simulink model "temperature"  (R2022a)
settings: Solver=VariableStepAuto  StartTime=0.0  StopTime=10.0  RelTol=1e-3
libraries: simulink x2, simulink_extras x1
settings Model: Creator=CTEA  LastModifiedBy=CTEA

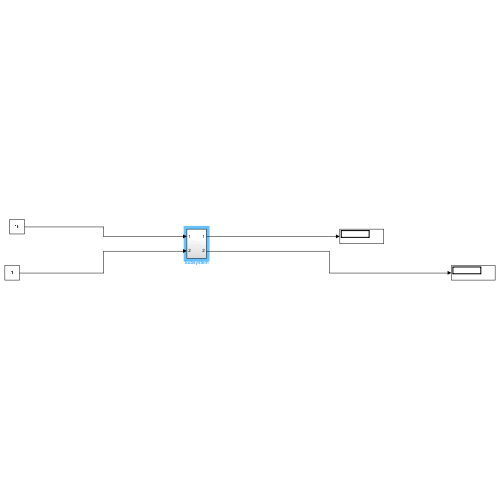
[thumbnail: Simulink's stored preview of the top-level diagram]
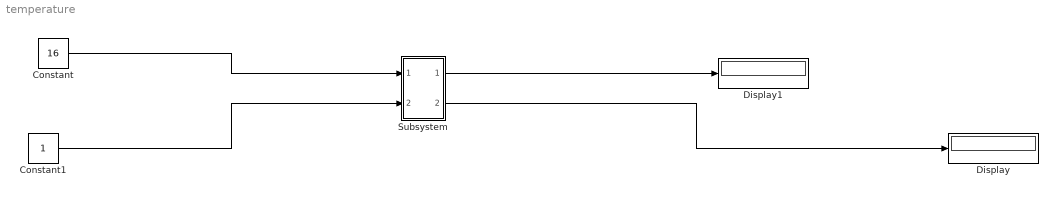
== system temperature ==
  Constant : Constant  Value=16  VectorParams1D=off
  Constant1 : Constant
  Display : Display
  Display1 : Display
  Subsystem : Subsystem
  wires:
  Constant/1 -> Subsystem/1(In1)
  Constant1/1 -> Subsystem/2(In2)
  Subsystem/2(Out1) -> Display/1
  Subsystem/1(Out2) -> Display1/1

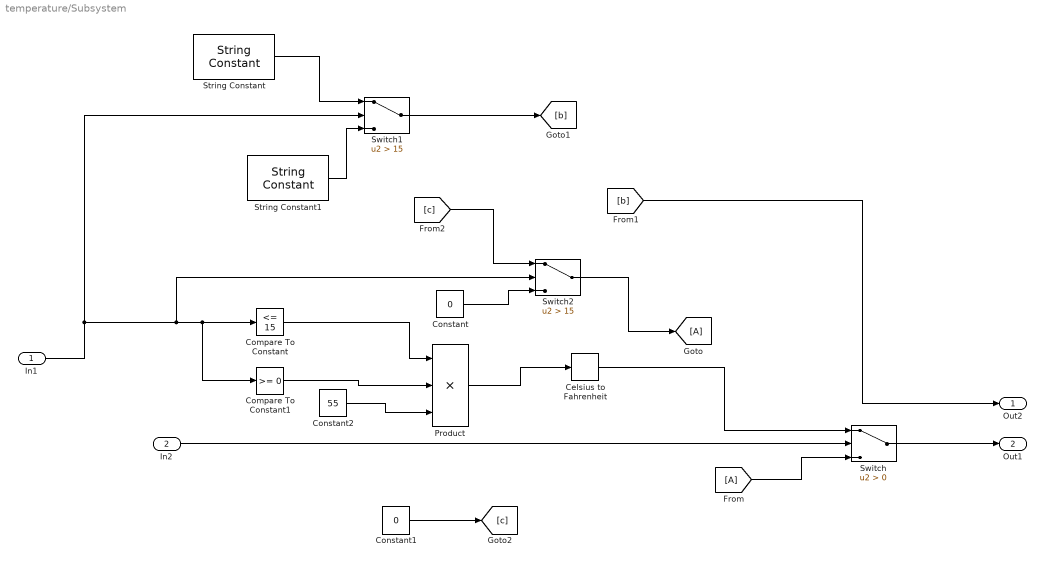
== system temperature/Subsystem ==
  In1 : Inport
  In2 : Inport  Port=2
  Celsius to Fahrenheit : simulink_extras/Transformations/Celsius to Fahrenheit
      settings: SourceProductBaseCode=SL
  Compare To Constant : simulink/Logic and Bit Operations/Compare To Constant  relop=<=  const=15  OutDataTypeStr=boolean
  Compare To Constant1 : simulink/Logic and Bit Operations/Compare To Constant  relop=>=  const=0  OutDataTypeStr=boolean
  Constant : Constant  Value=0
  Constant1 : Constant  Value=0
  Constant2 : Constant  Value=55
  From : From
  Goto : Goto
  Product : Product  Inputs=3
  String Constant : StringConstant  String="\"invalid\""
  String Constant1 : StringConstant  String="\"working\""
  Switch : Switch  Criteria=u2 > Threshold  SaturateOnIntegerOverflow=off  InputSameDT=off
  Switch1 : Switch  Criteria=u2 > Threshold  Threshold=15  SaturateOnIntegerOverflow=off  InputSameDT=off
  Switch2 : Switch  Criteria=u2 > Threshold  Threshold=15  SaturateOnIntegerOverflow=off  InputSameDT=off
  Out2 : Outport
  Out1 : Outport  Port=2
  wires:
  Product/1 -> Celsius to Fahrenheit/1
  In2/1 -> Switch/2
  Switch/1 -> Out1/1
  Celsius to Fahrenheit/1 -> Switch/1
  From/1 -> Switch/3
  Constant2/1 -> Product/3
  Compare To Constant/1 -> Product/1
  Compare To Constant1/1 -> Product/2
  String Constant/1 -> Switch1/1
  Switch1/1 -> [b]
  [b] -> Out2/1
  String Constant1/1 -> Switch1/3
  In1/1 -> Switch2/2, Compare To Constant1/1, Compare To Constant/1, Switch1/2
  Switch2/1 -> Goto/1
  Constant/1 -> Switch2/3
  [c] -> Switch2/1
  Constant1/1 -> [c]
